simulink model "AM_modulation"  (R2013a)
settings: Solver=ode45  StartTime=0.0  StopTime=200.0  RelTol=1e-3
settings Model: Creator=root  LastModifiedBy=root

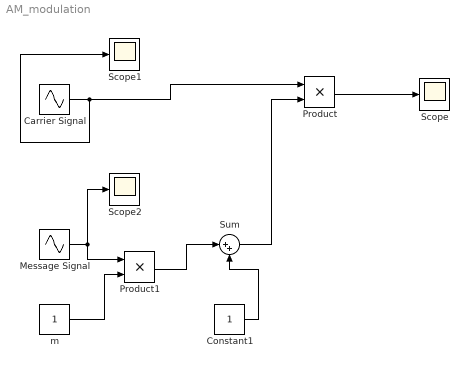
== system AM_modulation ==
  Carrier Signal : Sin  Frequency=2*pi*25  SampleTime=1/5000
  Constant1 : Constant
  Message Signal : Sin  Frequency=2*pi  SampleTime=1/5000
  Product : Product
  Product1 : Product
  Scope : Scope
  Scope1 : Scope
  Scope2 : Scope
      settings: SaveName=ScopeData2
  Sum : Sum  Inputs=|++
  m : Constant
  wires:
  Sum/1 -> Product/2
  Carrier Signal/1 -> Scope1/1, Product/1
  Message Signal/1 -> Scope2/1, Product1/1
  Constant1/1 -> Sum/2
  m/1 -> Product1/2
  Product1/1 -> Sum/1
  Product/1 -> Scope/1
